simulink subsystem "Gleichstrommaschine"  (R2022b)
settings: Solver=VariableStepAuto  StartTime=0.0  StopTime=10.0  RelTol=1e-3
values from neighbouring files (symbols this model uses):
  L_A = 0.11*10^-3    (= 0.00011)    [V4_Parameter_EM.m]    (also in V4_Parameter_Parameter_komplett_te.m; V4_Parameter_komplett.m)
  R_A = 0.36    [V4_Parameter_EM.m]    (also in V4_Parameter_Parameter_komplett_te.m; V4_Parameter_komplett.m)
settings Model: Creator=JSCHB  LastModifiedBy=JSCHB

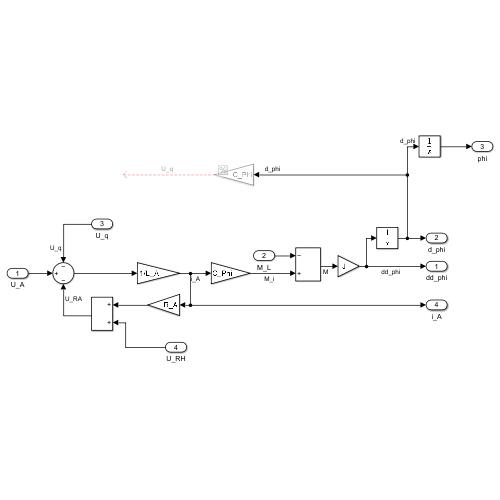
[thumbnail: Simulink's stored preview of the top-level diagram]
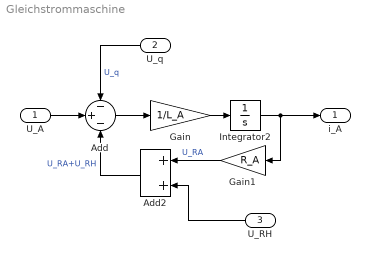
== system Gleichstrommaschine ==
  U_A : Inport
  U_q : Inport  Port=2
  U_RH : Inport  Port=3
  Add : Sum  Inputs=-+-
  Add2 : Sum
  Gain : Gain  Gain=1/L_A
  Gain1 : Gain  Gain=R_A
  Integrator2 : Integrator
  i_A : Outport
  wires:
  U_A/1 -> Add/2
  Add/1 -> Gain/1
  Gain/1 -> Integrator2/1
  Gain1/1 -> Add2/1  "U_RA"
  U_q/1 -> Add/1  "U_q"
  Add2/1 -> Add/3  "U_RA+U_RH"
  U_RH/1 -> Add2/2
  Integrator2/1 -> i_A/1, Gain1/1
